simulink model "sort_dutycycles"  (R2017b)
settings: Solver=FixedStepAuto  StartTime=0.0  StopTime=inf  RelTol=1e-3
PostLoadFcn:
  | , if any(exist('dsrtsu_mdlpostloadfcn', 'file') == [2, 3, 6]), try dsrtsu_mdlpostloadfcn('Execute', bdroot); catch fprintf('Error in PostLoadFcn (dsrtsu_mdlpostloadfcn) for model "%s":\n %s\n', bdroot, lasterr); end, end,
settings Model: DSRTSU_INTERNAL_RTI_VER=510  DSRTSU_INTERNAL_RTI_TYPE=rti1202  Creator=Z634594  LastModifiedBy=Z634594
settings HardwareCC: ProdBitPerPointer=32  ProdBitPerSizeT=32  ProdBitPerPtrDiffT=32  ProdLargestAtomicInteger=Integer  ProdEndianess=BigEndian  ProdWordSize=32  ProdHWDeviceType=Custom Processor->Custom  TargetIntDivRoundTo=Zero  TargetEndianess=BigEndian  TargetHWDeviceType=Custom Processor->Custom
settings SFSimCC: MATLABDynamicMemAlloc=off
settings RTWCC: SystemTargetFile=rti1202.tlc  MakeCommand=make_rti  TemplateMakefile=rti1202.tmf  Description=dSPACE DS1202 Hardware Platform
settings STFCustomTargetCC: ParMdlRefBuildCompliant=on  MatFileLogging=on  GRTInterface=off  SystemTargetFile=rti1202.tlc
settings GRTTargetCC: TargetLangStandard=C89/C90 (ANSI)  CompOptLevelCompliant=off  ConcurrentExecutionCompliant=off  CombineOutputUpdateFcns=off  CPPClassGenCompliant=off  UseToolchainInfoCompliant=off

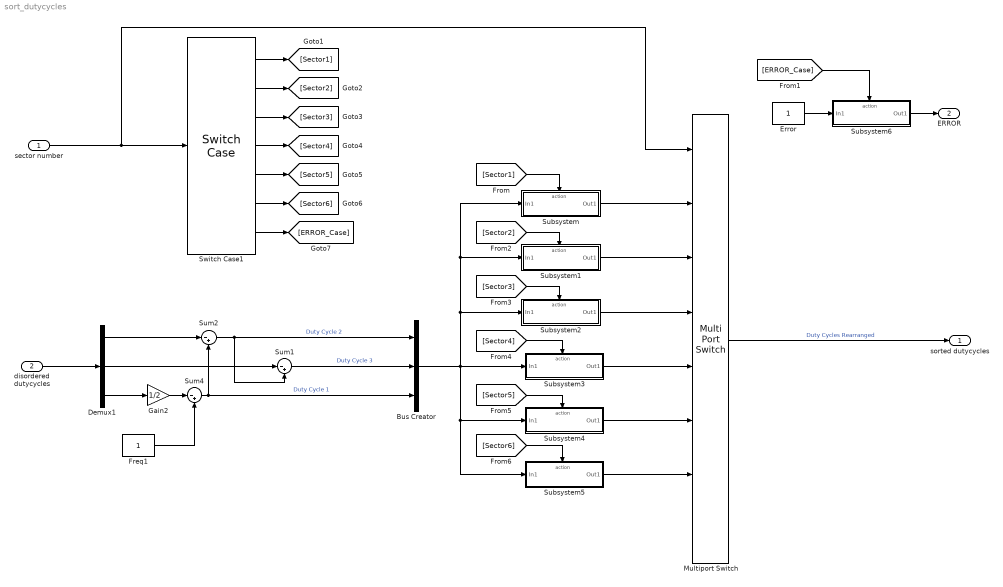
== system sort_dutycycles ==
  sector number : Inport
  disordered dutycycles : Inport  Port=2
  Bus Creator : BusCreator  Inputs=3
  Demux1 : Demux  Outputs=3
  Error : Constant
  Freq1 : Constant
  Gain2 : Gain  Gain=1/2
  Multiport Switch : MultiPortSwitch  Inputs=7
  Subsystem : Subsystem
  Subsystem1 : Subsystem
  Subsystem2 : Subsystem
  Subsystem3 : Subsystem
  Subsystem4 : Subsystem
  Subsystem5 : Subsystem
  Subsystem6 : Subsystem
  Sum1 : Sum  Inputs=|-+
  Sum2 : Sum  Inputs=|-+
  Sum4 : Sum  Inputs=|-+
  Switch Case1 : SwitchCase  CaseConditions={1,2,3,4,5,6}
  sorted dutycycles : Outport
  ERROR : Outport  Port=2
  wires:
  Gain2/1 -> Sum4/1
  sector number/1 -> Multiport Switch/1, Switch Case1/1
  Switch Case1/7 -> [ERROR_Case]
  Bus Creator/1 -> Subsystem/1(In1), Subsystem1/1(In1), Subsystem2/1(In1), Subsystem5/1(In1), Subsystem4/1(In1), Subsystem3/1(In1)
  Subsystem3/1(Out1) -> Multiport Switch/5
  Subsystem2/1(Out1) -> Multiport Switch/4
  Demux1/3 -> Gain2/1
  Multiport Switch/1 -> sorted dutycycles/1  "Duty Cycles Rearranged"
  Switch Case1/5 -> [Sector5]
  Subsystem4/1(Out1) -> Multiport Switch/6
  Switch Case1/3 -> [Sector3]
  Demux1/1 -> Sum2/1
  Sum2/1 -> Bus Creator/1, Sum1/2  "Duty Cycle 2"
  Sum1/1 -> Bus Creator/2  "Duty Cycle 3"
  [Sector1] -> Subsystem/Action
  [Sector3] -> Subsystem2/Action
  [Sector4] -> Subsystem3/Action
  Subsystem1/1(Out1) -> Multiport Switch/3
  [Sector2] -> Subsystem1/Action
  Demux1/2 -> Sum1/1
  disordered dutycycles/1 -> Demux1/1
  Freq1/1 -> Sum4/2
  Switch Case1/6 -> [Sector6]
  Switch Case1/2 -> [Sector2]
  Switch Case1/4 -> [Sector4]
  [Sector6] -> Subsystem5/Action
  Sum4/1 -> Bus Creator/3, Sum2/2  "Duty Cycle 1"
  Subsystem5/1(Out1) -> Multiport Switch/7
  [Sector5] -> Subsystem4/Action
  Switch Case1/1 -> [Sector1]
  Subsystem/1(Out1) -> Multiport Switch/2
  [ERROR_Case] -> Subsystem6/Action
  Subsystem6/1(Out1) -> ERROR/1
  Error/1 -> Subsystem6/1(In1)

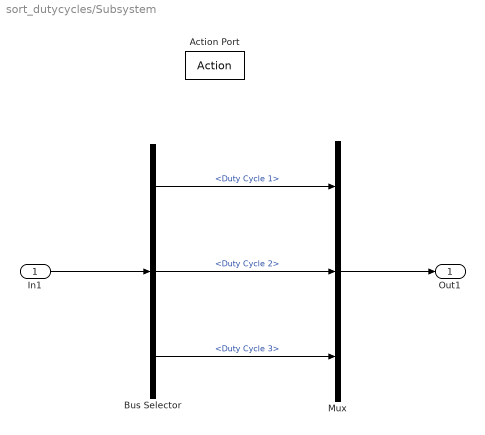
== system sort_dutycycles/Subsystem ==
  In1 : Inport
  Action Port : ActionPort  ActionType=case
  Bus Selector : BusSelector  OutputSignals=Duty Cycle 1,Duty Cycle 2,Duty Cycle 3
  Mux : Mux  Inputs=3
  Out1 : Outport
  wires:
  Mux/1 -> Out1/1
  Bus Selector/1 -> Mux/1  "<Duty Cycle 1>"
  Bus Selector/2 -> Mux/2  "<Duty Cycle 2>"
  Bus Selector/3 -> Mux/3  "<Duty Cycle 3>"
  In1/1 -> Bus Selector/1

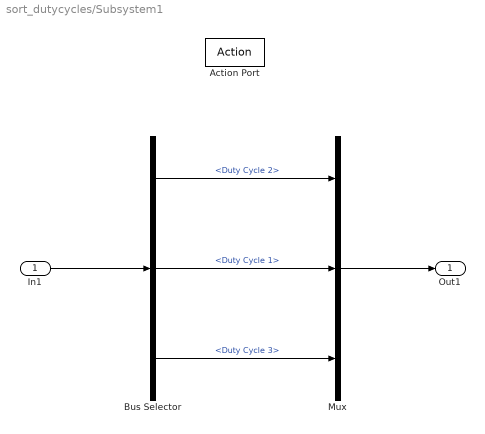
== system sort_dutycycles/Subsystem1 ==
  In1 : Inport
  Action Port : ActionPort  ActionType=case
  Bus Selector : BusSelector  OutputSignals=Duty Cycle 2,Duty Cycle 1,Duty Cycle 3
  Mux : Mux  Inputs=3
  Out1 : Outport
  wires:
  In1/1 -> Bus Selector/1
  Bus Selector/3 -> Mux/3  "<Duty Cycle 3>"
  Bus Selector/2 -> Mux/2  "<Duty Cycle 1>"
  Bus Selector/1 -> Mux/1  "<Duty Cycle 2>"
  Mux/1 -> Out1/1

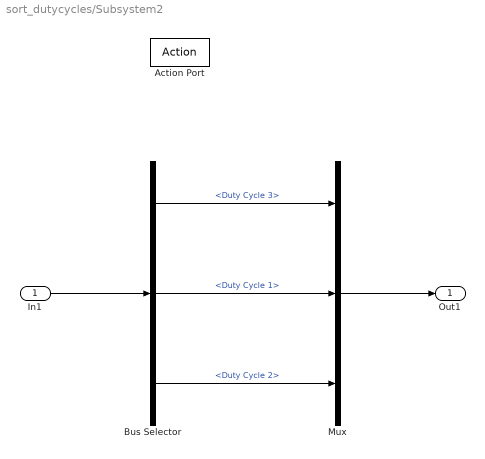
== system sort_dutycycles/Subsystem2 ==
  In1 : Inport
  Action Port : ActionPort  ActionType=case
  Bus Selector : BusSelector  OutputSignals=Duty Cycle 3,Duty Cycle 1,Duty Cycle 2
  Mux : Mux  Inputs=3
  Out1 : Outport
  wires:
  Bus Selector/3 -> Mux/3  "<Duty Cycle 2>"
  Bus Selector/1 -> Mux/1  "<Duty Cycle 3>"
  Mux/1 -> Out1/1
  Bus Selector/2 -> Mux/2  "<Duty Cycle 1>"
  In1/1 -> Bus Selector/1

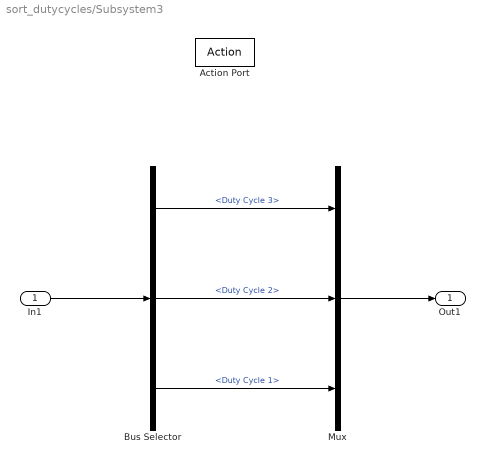
== system sort_dutycycles/Subsystem3 ==
  In1 : Inport
  Action Port : ActionPort  ActionType=case
  Bus Selector : BusSelector  OutputSignals=Duty Cycle 3,Duty Cycle 2,Duty Cycle 1
  Mux : Mux  Inputs=3
  Out1 : Outport
  wires:
  Bus Selector/3 -> Mux/3  "<Duty Cycle 1>"
  Bus Selector/2 -> Mux/2  "<Duty Cycle 2>"
  In1/1 -> Bus Selector/1
  Mux/1 -> Out1/1
  Bus Selector/1 -> Mux/1  "<Duty Cycle 3>"

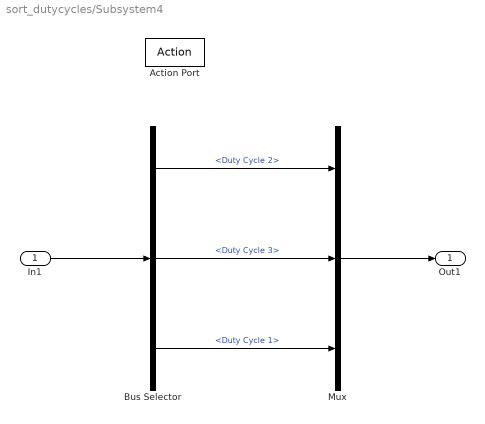
== system sort_dutycycles/Subsystem4 ==
  In1 : Inport
  Action Port : ActionPort  ActionType=case
  Bus Selector : BusSelector  OutputSignals=Duty Cycle 2,Duty Cycle 3,Duty Cycle 1
  Mux : Mux  Inputs=3
  Out1 : Outport
  wires:
  Bus Selector/2 -> Mux/2  "<Duty Cycle 3>"
  Bus Selector/1 -> Mux/1  "<Duty Cycle 2>"
  Mux/1 -> Out1/1
  In1/1 -> Bus Selector/1
  Bus Selector/3 -> Mux/3  "<Duty Cycle 1>"

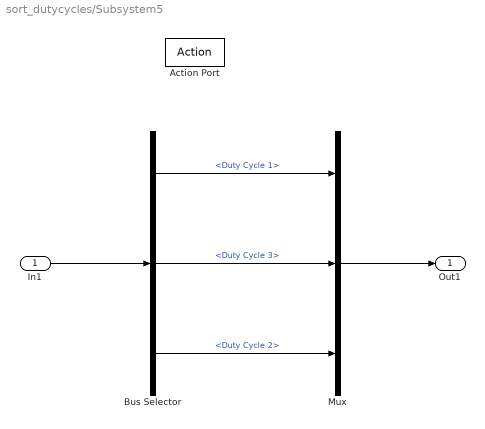
== system sort_dutycycles/Subsystem5 ==
  In1 : Inport
  Action Port : ActionPort  ActionType=case
  Bus Selector : BusSelector  OutputSignals=Duty Cycle 1,Duty Cycle 3,Duty Cycle 2
  Mux : Mux  Inputs=3
  Out1 : Outport
  wires:
  Bus Selector/3 -> Mux/3  "<Duty Cycle 2>"
  Bus Selector/1 -> Mux/1  "<Duty Cycle 1>"
  Bus Selector/2 -> Mux/2  "<Duty Cycle 3>"
  In1/1 -> Bus Selector/1
  Mux/1 -> Out1/1

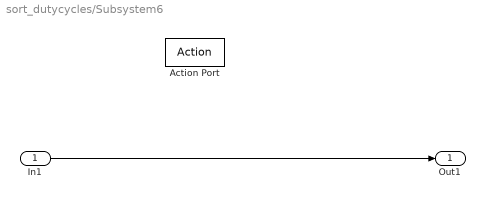
== system sort_dutycycles/Subsystem6 ==
  In1 : Inport
  Action Port : ActionPort  ActionType=default
  Out1 : Outport
  wires:
  In1/1 -> Out1/1
